simulink model "LCK"  (R2018b)
settings: Solver=FixedStepDiscrete  StartTime=0.0  StopTime=inf  FixedStep=0.01  RelTol=1e-3
PostLoadFcn:
  | if any(exist('dsrtsu_mdlpostloadfcn', 'file') ~= 0), dsrtsu_mdlpostloadfcn('Execute', bdroot); end
values from neighbouring files (symbols this model uses):
  C_DEG2RAD = 0.0175    [LCK_Macro.sldd]
  C_KPH2MPS = 0.2778    [LCK_Macro.sldd]
  C_NEARZERO = 0.0001    [LCK_Macro.sldd]
  C_ONE = 1.0    [LCK_Macro.sldd]
  C_RAD2DEG = 57.2958    [LCK_Macro.sldd]
  C_ZERO = 0.0    [LCK_Macro.sldd]
  k_accel_pedal_pos_per_speed_x : value not decoded    [LCK_LogicPara.sldd]
  k_accel_pedal_pos_per_speed_z : value not decoded    [LCK_LogicPara.sldd]
  k_brake_suprress_hold = 1000.0    [LCK_LogicPara.sldd]
  k_driver_appl_torque_filt = 50.0    [LCK_LogicPara.sldd]
  k_driver_suppression_hold_time = 3000.0    [LCK_LogicPara.sldd]
  k_hands_on_wheel_hold_msec = 500.0    [LCK_LogicPara.sldd]
  k_hands_on_wheel_torque_hi = 0.2    [LCK_LogicPara.sldd]
  k_hands_on_wheel_torque_lo = 0.15    [LCK_LogicPara.sldd]
  k_handsoff_delay_cycles = 50.0    [LCK_LogicPara.sldd]
  k_handsoff_torq_Lo_CR = 0.3    [LCK_LogicPara.sldd]
  k_handson_delay_cycles = 5.0    [LCK_LogicPara.sldd]
  k_HighAccel_suppress_hold = 3000.0    [LCK_LogicPara.sldd]
  k_HLR_suprress_hold = 3000.0    [LCK_LogicPara.sldd]
  k_hs_StrAng_CR_threshold_z : value not decoded    [LCK_LogicPara.sldd]
  k_LC_Exit_Switch = 0.0    [LCK_LogicPara.sldd]
  k_LCG_Configured = 1.0    [LCK_LogicPara.sldd]
  k_LCK_A0_Rdy2Act_UseConst = 0.0    [LCK_LogicPara.sldd]
  k_LCK_A0Fac_ActSta : value not decoded    [LCK_CtrlPara.sldd]
  k_LCK_A0Fac_DrvStm : value not decoded    [LCK_CtrlPara.sldd]
  k_LCK_A0Shift_LftCurv : value not decoded    [LCK_CtrlPara.sldd]
  k_LCK_A0Shift_RgtCurv : value not decoded    [LCK_CtrlPara.sldd]
  k_LCK_A0Shift_StraLan = 0.0    [LCK_CtrlPara.sldd]
  k_LCK_A0ShiftFac_Dy_LftCurv : value not decoded    [LCK_CtrlPara.sldd]
  k_LCK_A0ShiftFac_Dy_RgtCurv : value not decoded    [LCK_CtrlPara.sldd]
  k_LCK_A0ShiftFac_Vspd : value not decoded    [LCK_CtrlPara.sldd]
  k_LCK_accel_inhibit_thold = 35.0    [LCK_LogicPara.sldd]
  k_LCK_Active2Ready_Mask = 255.0    [LCK_LogicPara.sldd]
  k_LCK_CvatRateBks : value not decoded    [LCK_CtrlPara.sldd]
  k_LCK_CvatrBks : value not decoded    [LCK_CtrlPara.sldd]
  k_LCK_DFac_Dy : value not decoded    [LCK_CtrlPara.sldd]
  k_LCK_DFac_Dy_Curv : value not decoded    [LCK_CtrlPara.sldd]
  k_LCK_DFac_HaCurCen : value not decoded    [LCK_CtrlPara.sldd]
  k_LCK_DFac_HaCurSid : value not decoded    [LCK_CtrlPara.sldd]
  k_LCK_DFac_HadCurCen : value not decoded    [LCK_CtrlPara.sldd]
  k_LCK_DFac_HadCurSid : value not decoded    [LCK_CtrlPara.sldd]
  k_LCK_DFac_HadStrCen : value not decoded    [LCK_CtrlPara.sldd]
  k_LCK_DFac_HadStrSid : value not decoded    [LCK_CtrlPara.sldd]
  k_LCK_DFac_HaStrCen : value not decoded    [LCK_CtrlPara.sldd]
  k_LCK_DFac_HaStrSid : value not decoded    [LCK_CtrlPara.sldd]
  k_LCK_DFac_Rad : value not decoded    [LCK_CtrlPara.sldd]
  k_LCK_DFac_SA_CurCen : value not decoded    [LCK_CtrlPara.sldd]
  k_LCK_DFac_SA_CurSid : value not decoded    [LCK_CtrlPara.sldd]
  k_LCK_DFac_SA_StrCen : value not decoded    [LCK_CtrlPara.sldd]
  k_LCK_DFac_SA_StrSid : value not decoded    [LCK_CtrlPara.sldd]
  k_LCK_DFac_SS_CurCen : value not decoded    [LCK_CtrlPara.sldd]
  k_LCK_DFac_SS_CurSid : value not decoded    [LCK_CtrlPara.sldd]
  k_LCK_DFac_SS_StrCen : value not decoded    [LCK_CtrlPara.sldd]
  k_LCK_DFac_SS_StrSid : value not decoded    [LCK_CtrlPara.sldd]
  k_LCK_DFac_Vspd : value not decoded    [LCK_CtrlPara.sldd]
  k_LCK_DlyTm_DrvStim = 0.2    [LCK_CtrlPara.sldd]
  k_LCK_DTermMax = 2.0    [LCK_CtrlPara.sldd]
  k_LCK_DyBks_Curv : value not decoded    [LCK_CtrlPara.sldd]
  k_LCK_Enable_POOnly = 1.0    [LCK_LogicPara.sldd]
  k_LCK_Entry_DistBuffer = 0.1    [LCK_LogicPara.sldd]
  k_LCK_Fac_Vspd2RngThr_FalRec = 0.23    [LCK_CtrlPara.sldd]
  k_LCK_Ffw_CvatSwh = 0.0    [LCK_CtrlPara.sldd]
  k_LCK_Ffw_DyBks : value not decoded    [LCK_CtrlPara.sldd]
  k_LCK_Ffw_TimCon_CmdFlt = 0.0    [LCK_CtrlPara.sldd]
  k_LCK_FfwDeltaFac_Rad_Lft : value not decoded    [LCK_CtrlPara.sldd]
  k_LCK_FfwDeltaFac_Rad_Rgt : value not decoded    [LCK_CtrlPara.sldd]
  k_LCK_FfwDeltaFac_Vspd : value not decoded    [LCK_CtrlPara.sldd]
  k_LCK_FfwFac_CvatRate_Lft : value not decoded    [LCK_CtrlPara.sldd]
  k_LCK_FfwFac_CvatRate_Rgt : value not decoded    [LCK_CtrlPara.sldd]
  k_LCK_FfwFac_Dy : value not decoded    [LCK_CtrlPara.sldd]
  k_LCK_FfwFac_Rad_Lft : value not decoded    [LCK_CtrlPara.sldd]
  k_LCK_FfwFac_Rad_Rgt : value not decoded    [LCK_CtrlPara.sldd]
  k_LCK_FfwFac_Vspd : value not decoded    [LCK_CtrlPara.sldd]
  k_LCK_FfwTorq_Cvat : value not decoded    [LCK_CtrlPara.sldd]
  k_LCK_HAFac_ActSta : value not decoded    [LCK_CtrlPara.sldd]
  k_LCK_HAFac_DrvStm : value not decoded    [LCK_CtrlPara.sldd]
  k_LCK_HaloTime = 2000.0    [LCK_LogicPara.sldd]
  k_LCK_HaloTime_Switch = 0.0    [LCK_LogicPara.sldd]
  k_LCK_HARFac_ActSta : value not decoded    [LCK_CtrlPara.sldd]
  k_LCK_HARFac_DrvStm : value not decoded    [LCK_CtrlPara.sldd]
  k_LCK_Hed_DyBks : value not decoded    [LCK_CtrlPara.sldd]
  k_LCK_HedAngDiffX : value not decoded    [LCK_CtrlPara.sldd]
  k_LCK_HedAngRateDiffX : value not decoded    [LCK_CtrlPara.sldd]
  k_LCK_HndsOnWhel_DlyTm_Idl2Rdy = 0.0    [LCK_LogicPara.sldd]
  k_LCK_host_veh_width = 1.86    [LCK_LogicPara.sldd]
  k_LCK_Idle2Ready_Mask = 239.0    [LCK_LogicPara.sldd]
  k_LCK_Junc_SusTime = 1.0    [LCK_LogicPara.sldd]
  k_LCK_KpKdDecSlopeLmt = 10.0    [LCK_CtrlPara.sldd]
  k_LCK_KpKdIncSlopeLmt = 5.0    [LCK_CtrlPara.sldd]
  k_LCK_Lat_Ctrl_DFac_Lft = 1.0    [LCK_CtrlPara.sldd]
  k_LCK_Lat_Ctrl_DFac_Rgt = 1.05    [LCK_CtrlPara.sldd]
  k_LCK_Lat_Ctrl_Kd = 0.8    [LCK_CtrlPara.sldd]
  k_LCK_Lat_Ctrl_Ki = 0.5    [LCK_CtrlPara.sldd]
  k_LCK_Lat_Ctrl_Kp = 0.7    [LCK_CtrlPara.sldd]
  k_LCK_Lat_Ctrl_Kp_NearGain = 0.7    [LCK_CtrlPara.sldd]
  k_LCK_Lat_Ctrl_PFac_Lft = 1.0    [LCK_CtrlPara.sldd]
  k_LCK_Lat_Ctrl_PFac_Rgt = 1.05    [LCK_CtrlPara.sldd]
  k_LCK_Lat_Ctrl_TimCon_CmdFlt = 5.0    [LCK_CtrlPara.sldd]
  k_LCK_Lat_DFac_Rad : value not decoded    [LCK_CtrlPara.sldd]
  k_LCK_Lat_DFac_SS_Cur : value not decoded    [LCK_CtrlPara.sldd]
  k_LCK_Lat_DFac_SS_Str : value not decoded    [LCK_CtrlPara.sldd]
  k_LCK_Lat_DFac_Vspd : value not decoded    [LCK_CtrlPara.sldd]
  k_LCK_Lat_DyBks : value not decoded    [LCK_CtrlPara.sldd]
  k_LCK_Lat_IFac_Rad : value not decoded    [LCK_CtrlPara.sldd]
  k_LCK_Lat_IFac_Vspd : value not decoded    [LCK_CtrlPara.sldd]
  k_LCK_Lat_ILmtFac_Dy_CurvLan : value not decoded    [LCK_CtrlPara.sldd]
  k_LCK_Lat_ILmtFac_Dy_StraLan : value not decoded    [LCK_CtrlPara.sldd]
  k_LCK_Lat_ILmtFac_Rad : value not decoded    [LCK_CtrlPara.sldd]
  k_LCK_Lat_ILmtFac_Rad_NearGain = 1.0    [LCK_CtrlPara.sldd]
  k_LCK_Lat_ILmtFac_Vspd_CurvLan : value not decoded    [LCK_CtrlPara.sldd]
  k_LCK_Lat_ILmtFac_Vspd_StraLan : value not decoded    [LCK_CtrlPara.sldd]
  k_LCK_Lat_ITermLmt_Dy = 1.0    [LCK_CtrlPara.sldd]
  k_LCK_Lat_KpKdDecSlopeLmt = 10.0    [LCK_CtrlPara.sldd]
  k_LCK_Lat_KpKdIncSlopeLmt = 10.0    [LCK_CtrlPara.sldd]
  k_LCK_Lat_PFac_Dy_InnLftCur : value not decoded    [LCK_CtrlPara.sldd]
  k_LCK_Lat_PFac_Dy_InnRgtCur : value not decoded    [LCK_CtrlPara.sldd]
  k_LCK_Lat_PFac_Dy_OutLftCur : value not decoded    [LCK_CtrlPara.sldd]
  k_LCK_Lat_PFac_Dy_OutRgtCur : value not decoded    [LCK_CtrlPara.sldd]
  k_LCK_Lat_PFac_Dy_Str : value not decoded    [LCK_CtrlPara.sldd]
  k_LCK_Lat_PFac_Rad : value not decoded    [LCK_CtrlPara.sldd]
  ... (+153 more)
undefined symbols (not defined in the file or in its folder): k_LCK_CurvBks, K_LCK_SPA0A1A2_LMRngCmp_y
libraries: LateralControl_fcns_lib x59, simulink x24
(part 17 of 47)

== system LCK/Lateral_Control_Module/Adas_Lateral_Control_LCK_Core/Module 10/Calculation of Feed Forward Torq ==
  Vspd : Inport
  Current_Dy : Inport  Port=2
  Curvat_Rat : Inport  Port=3
  Curvature_0 : Inport  Port=4
  Curvature_1 : Inport  Port=5
  Road_Radius : Inport  Port=6
  Abs : Abs
  Abs1 : Abs
  Add : Sum
  Compare To Zero2 : simulink/Logic and Bit Operations/Compare To Zero  relop=<=  OutDataTypeStr=boolean
  Compare To Zero3 : simulink/Logic and Bit Operations/Compare To Zero  relop=<=  OutDataTypeStr=boolean
  Compare To Zero4 : simulink/Logic and Bit Operations/Compare To Zero  relop=<=  OutDataTypeStr=boolean
  Gain : Gain  Gain=-1
  Gain1 : Gain  Gain=-1
  Product2 : Product  Inputs=5
  Product3 : Product  Inputs=5
  Sign : Signum
  Sign1 : Signum
  Switch{1,6..8} (4 alike) : Switch  Criteria=u2 > Threshold
  k_LCK_FfwDeltaFac_Rad_Lft : Lookup_n-D  NumberOfTableDimensions=1  BreakpointsForDimension1=k_LCK_RadBks  BreakpointsForDimension2=k_LCK_CurvBks  IndexSearchMethod=Linear search  Table=k_LCK_FfwDeltaFac_Rad_Lft  ExtrapMethod=Clip  InternalRulePriority=Speed  RndMeth=Simplest  InputSameDT=on
  k_LCK_FfwDeltaFac_Rad_Rgt : Lookup_n-D  NumberOfTableDimensions=1  BreakpointsForDimension1=k_LCK_RadBks  BreakpointsForDimension2=k_LCK_CurvBks  IndexSearchMethod=Linear search  Table=k_LCK_FfwDeltaFac_Rad_Rgt  ExtrapMethod=Clip  InternalRulePriority=Speed  RndMeth=Simplest  InputSameDT=on
  k_LCK_FfwDeltaFac_Vspd : Lookup_n-D  NumberOfTableDimensions=1  BreakpointsForDimension1=k_LCK_VspdBks  BreakpointsForDimension2=k_LCK_CurvBks  IndexSearchMethod=Linear search  Table=k_LCK_FfwDeltaFac_Vspd  ExtrapMethod=Clip  InternalRulePriority=Speed  RndMeth=Simplest  InputSameDT=on
  k_LCK_FfwFac_CvatRate_Lft : Lookup_n-D  NumberOfTableDimensions=1  BreakpointsForDimension1=k_LCK_CvatRateBks  BreakpointsForDimension2=k_LCK_CurvBks  IndexSearchMethod=Linear search  Table=k_LCK_FfwFac_CvatRate_Lft  ExtrapMethod=Clip  InternalRulePriority=Speed  RndMeth=Simplest  InputSameDT=on
  k_LCK_FfwFac_CvatRate_Rgt : Lookup_n-D  NumberOfTableDimensions=1  BreakpointsForDimension1=k_LCK_CvatRateBks  BreakpointsForDimension2=k_LCK_CurvBks  IndexSearchMethod=Linear search  Table=k_LCK_FfwFac_CvatRate_Rgt  ExtrapMethod=Clip  InternalRulePriority=Speed  RndMeth=Simplest  InputSameDT=on
  k_LCK_FfwFac_Dy : Lookup_n-D  NumberOfTableDimensions=1  BreakpointsForDimension1=k_LCK_Ffw_DyBks  BreakpointsForDimension2=k_LCK_CurvBks  IndexSearchMethod=Linear search  Table=k_LCK_FfwFac_Dy  ExtrapMethod=Clip  InternalRulePriority=Speed  RndMeth=Simplest  InputSameDT=on
  k_LCK_FfwFac_Rad_Lft : Lookup_n-D  NumberOfTableDimensions=1  BreakpointsForDimension1=k_LCK_RadBks  BreakpointsForDimension2=k_LCK_CurvBks  IndexSearchMethod=Linear search  Table=k_LCK_FfwFac_Rad_Lft  ExtrapMethod=Clip  InternalRulePriority=Speed  RndMeth=Simplest  InputSameDT=on
  k_LCK_FfwFac_Rad_Rgt : Lookup_n-D  NumberOfTableDimensions=1  BreakpointsForDimension1=k_LCK_RadBks  BreakpointsForDimension2=k_LCK_CurvBks  IndexSearchMethod=Linear search  Table=k_LCK_FfwFac_Rad_Rgt  ExtrapMethod=Clip  InternalRulePriority=Speed  RndMeth=Simplest  InputSameDT=on
  k_LCK_FfwFac_Vspd : Lookup_n-D  NumberOfTableDimensions=1  BreakpointsForDimension1=k_LCK_VspdBks  BreakpointsForDimension2=k_LCK_CurvBks  IndexSearchMethod=Linear search  Table=k_LCK_FfwFac_Vspd  ExtrapMethod=Clip  InternalRulePriority=Speed  RndMeth=Simplest  InputSameDT=on
  k_LCK_FfwTorq_Cvat : Lookup_n-D  NumberOfTableDimensions=1  BreakpointsForDimension1=k_LCK_CvatrBks  BreakpointsForDimension2=k_LCK_CurvBks  IndexSearchMethod=Linear search  Table=k_LCK_FfwTorq_Cvat  ExtrapMethod=Clip  InternalRulePriority=Speed  RndMeth=Simplest  InputSameDT=on
  k_LCK_Ffw_CvatSwh : Constant  Description=_GWMAB30P3.LCK.000_154_  Value=k_LCK_Ffw_CvatSwh
  FfwFac_CvatRate : Outport
  FfwFac_Dy : Outport  Port=2
  FfwTorq_Basic : Outport  Port=3
  FfwTorq_Delta : Outport  Port=4
  Feed_Forward_Torq : Outport  Port=5
  wires:
  [Curvature] -> Compare To Zero2/1
  Compare To Zero2/1 -> Switch6/2
  k_LCK_FfwDeltaFac_Vspd/1 -> Product3/3
  Road_Radius/1 -> k_LCK_FfwFac_Rad_Lft/1, k_LCK_FfwFac_Rad_Rgt/1, k_LCK_FfwDeltaFac_Rad_Lft/1, k_LCK_FfwDeltaFac_Rad_Rgt/1
  Compare To Zero3/1 -> Switch1/2
  Add/1 -> Feed_Forward_Torq/1
  k_LCK_FfwFac_Vspd/1 -> Product2/4
  Product2/1 -> Add/1, FfwTorq_Basic/1
  Sign1/1 -> Product3/5
  Gain1/1 -> Sign1/1
  Product3/1 -> FfwTorq_Delta/1, Add/2
  [Vspd] -> k_LCK_FfwDeltaFac_Vspd/1
  k_LCK_FfwFac_Dy/1 -> FfwFac_Dy/1, Product3/1
  k_LCK_FfwTorq_Cvat/1 -> [FfwTorq_Cvat], Product2/1
  Switch6/1 -> Product2/3
  [Curvature] -> Compare To Zero4/1
  Current_Dy/1 -> [Dy], Abs/1
  Abs/1 -> k_LCK_FfwFac_Dy/1
  Abs1/1 -> k_LCK_FfwTorq_Cvat/1
  k_LCK_FfwFac_CvatRate_Lft/1 -> Switch1/1
  k_LCK_FfwFac_CvatRate_Rgt/1 -> Switch1/3
  k_LCK_FfwFac_Rad_Lft/1 -> Switch6/1
  Vspd/1 -> [Vspd], k_LCK_FfwFac_Vspd/1
  Curvat_Rat/1 -> k_LCK_FfwFac_CvatRate_Rgt/1, k_LCK_FfwFac_CvatRate_Lft/1
  Curvature_1/1 -> Switch8/3
  Curvature_0/1 -> Switch8/1
  k_LCK_Ffw_CvatSwh/1 -> Switch8/2
  k_LCK_FfwDeltaFac_Rad_Lft/1 -> Switch7/1
  k_LCK_FfwDeltaFac_Rad_Rgt/1 -> Switch7/3
  [Curvature] -> Compare To Zero3/1
  Compare To Zero4/1 -> Switch7/2
  Switch8/1 -> [Curvature], Abs1/1
  k_LCK_FfwFac_Rad_Rgt/1 -> Switch6/3
  Switch7/1 -> Product3/2
  Gain/1 -> Sign/1
  Sign/1 -> Product2/5
  [Dy] -> Gain1/1
  [Curvature] -> Gain/1
  Switch1/1 -> Product2/2, FfwFac_CvatRate/1
  [FfwTorq_Cvat] -> Product3/4

== system LCK/Lateral_Control_Module/Adas_Lateral_Control_LCK_Core/Module 11/Non-Linear Compenastion ==
  Lat_Ctrl_Cmd : Inport
  LatCtrl_Cmd : Inport  Port=2
  Ffw_Ctrl_Cmd : Inport  Port=3
  SPPRecognition_Type : Inport  Port=4
  Vspd : Inport  Port=5
  Abs : Abs
  Constant1 : Constant  Tag={'output',{'name','$P','class','EXTERN_MACRO','type','ESR_Typedefs/unsigned8_T'},'date',737462.69417376153}  Description=_GWMH9P4.LCK.000_202_  Value=0  OutDataTypeStr=single
  Constant2 : Constant  Tag={'output',{'name','$P','class','EXTERN_MACRO','type','ESR_Typedefs/unsigned8_T'},'date',737462.69417376153}  Description=_GWMH9P4.LCK.000_202_  Value=2  OutDataTypeStr=uint8
  Constant3 : Constant  Tag={'output',{'name','$P','class','EXTERN_MACRO','type','ESR_Typedefs/unsigned8_T'},'date',737462.69417376153}  Description=_GWMH9P4.LCK.000_202_  Value=0
  Divide : Product  Inputs=*/
  Product3 : Product  Inputs=3  RndMeth=Zero
  Relational Operator3 : RelationalOperator  Operator=<=  OutDataTypeStr=boolean  RndMeth=Nearest
  Saturation1 : Saturate  UpperLimit=3  LowerLimit=-3  OutDataTypeStr=Inherit: Inherit via back propagation
  Sum1 : Sum  Description=_GWMAB30P2.LCK.000_1363_
  Sum2 : Sum  Description=_GWMAB30P2.LCK.000_1363_  Inputs=+++
  Switch1 : Switch  Description=_GWMAB30P2.LCK.000_1368_  Threshold=0.5
  Switch10 : Switch  Description=_GWMAB30P2.LCK.000_1368_  Threshold=0.5
  Switch3 : Switch  Description=_GWMAB30P2.LCK.000_1368_  Threshold=0.5
  k_LCK_NonLinCompFac_Vspd : Lookup_n-D  NumberOfTableDimensions=1  BreakpointsForDimension1=k_LCK_VspdBks  IndexSearchMethod=Linear search  Table=k_LCK_NonLinCompFac_Vspd  ExtrapMethod=Clip  InternalRulePriority=Speed  RndMeth=Simplest  InputSameDT=on
  k_LCK_NonLinCompTab : Lookup_n-D  NumberOfTableDimensions=1  BreakpointsForDimension1=k_LCK_TorqCmdBks  IndexSearchMethod=Linear search  Table=k_LCK_NonLinCompTab  ExtrapMethod=Clip  InternalRulePriority=Speed  RndMeth=Simplest  InputSameDT=on
  k_LCK_NonLinearComp_En : Constant  Description=_GWMAB30P3.LCK.000_168_  Value=k_LCK_NonLinearComp_En
  LCK_PIDTorqCmd : Outport
  LCK_PIDPlusFfw_TorqCmd : Outport  Port=2
  LCK_PIDTorqCmd_Percent : Outport  Port=3
  LCK_TorqCmd_Cmpd : Outport  Port=4
  wires:
  k_LCK_NonLinearComp_En/1 -> Switch3/2
  Switch3/1 -> Saturation1/1
  Ffw_Ctrl_Cmd/1 -> Sum2/3
  Lat_Ctrl_Cmd/1 -> Sum1/1, Sum2/1
  LatCtrl_Cmd/1 -> Sum1/2, Sum2/2
  Vspd/1 -> k_LCK_NonLinCompFac_Vspd/1
  Abs/1 -> k_LCK_NonLinCompTab/1
  k_LCK_NonLinCompTab/1 -> Product3/2
  k_LCK_NonLinCompFac_Vspd/1 -> Product3/3
  Saturation1/1 -> LCK_TorqCmd_Cmpd/1
  Product3/1 -> Switch3/1
  SPPRecognition_Type/1 -> Relational Operator3/1
  Constant2/1 -> Relational Operator3/2
  Relational Operator3/1 -> Switch10/2, Switch1/2
  Sum2/1 -> Switch10/1
  Constant1/1 -> Switch10/3
  Switch10/1 -> LCK_PIDPlusFfw_TorqCmd/1, Switch3/3, Divide/2, Product3/1, Abs/1
  Sum1/1 -> Switch1/1
  Constant3/1 -> Switch1/3
  Switch1/1 -> Divide/1, LCK_PIDTorqCmd/1
  Divide/1 -> LCK_PIDTorqCmd_Percent/1
